simulink model "TransitionPriorities"  (Simulink 7.4)
settings: Solver=ode45  StartTime=0.0  StopTime=10.0  RelTol=1e-3
settings Model: Creator=dread  LastModifiedBy=dread

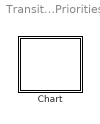
== system TransitionPriorities ==
  Chart : Stateflow chart

== stateflow chart Chart ==
  state A
  state B
  A -> B [order 1] : [Prio1]
  A -> B [order 2] : [Prio2]
  A -> B [order 3] : [Prio3]
